simulink model "RotaryPendulum_SLdemo_SwingUp"  (R2015a)
settings: Solver=ode45  StartTime=0.0  StopTime=30  MaxStep=1e-3
InitFcn:
  | RotaryPendulum_PARAM;
values from neighbouring files (symbols this model uses):
  R = 0    [RotaryPendulum_MLdemo.m]
undefined symbols (not defined in the file or in its folder): g, I, l, m
libraries: vrlib x1, aerolibanimutils x1
settings Model: CovSFcnEnable=off  Creator=mischak  LastModifiedBy=mischak
settings DebuggingCC: SolverPrmCheckMsg=warning

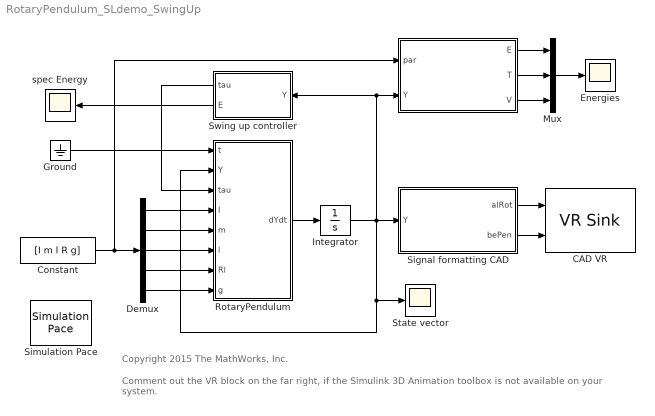
== system RotaryPendulum_SLdemo_SwingUp ==
  note: Comment out the VR block on the far right, if the Simulink 3D Animation toolbox is not available on your system.
  note: Copyright 2015 The MathWorks, Inc.
  " " : MATLAB Function  TreatAsAtomicUnit=on
  CAD VR : vrlib/VR Sink  InstantiateOnLoad=on  SampleTime=0.1  ViewEnable=on  RemoteChange=off  RemoteView=off  FieldsWritten=BFrame.rotation.4.1.1.double#EFrame.rotation.4.1.1.double  WorldFileName=SolidWorksS3D.wrl  AutoView=off  VideoDimensions=[]  AllowVariableSize=off  mask(Virtual Reality Sink){}
      mask Display: image(imread('SolidWorksS3D_icon.png'))
  Constant : Constant  Value=[I m l R g]
  Demux : Demux  Outputs=5
  Energies : Scope
      settings: YMin=-0.003  YMax=0.006
  Ground : Ground
  Integrator : Integrator  InitialCondition=[0 0 3.2 0.2]
  Mux : Mux  Inputs=3
  RotaryPendulum : MATLAB Function  TreatAsAtomicUnit=on
  Signal formatting CAD : MATLAB Function  TreatAsAtomicUnit=on
  Simulation Pace : aerolibanimutils/Simulation Pace  SimulationPace=0.75  SleepMode=MATLAB Thread  OutputPaceError=off  SampleTime=1/20
      settings: AttributesFormatString=%<SimulationPace> sec/sec
  State vector : Scope
      settings: YMin=-12.5  YMax=12.5
  Swing up controller : MATLAB Function  TreatAsAtomicUnit=on
  spec Energy : Scope
      settings: YMin=-2.1  YMax=-1.9  SaveName=ScopeData3
  wires:
  Integrator/1 -> Signal formatting CAD/1(Y), RotaryPendulum/2(Y), State vector/1, " "/2(Y), Swing up controller/1(Y)
  RotaryPendulum/1(dYdt) -> Integrator/1
  Demux/1 -> RotaryPendulum/4(I)
  Demux/3 -> RotaryPendulum/6(l)
  Demux/4 -> RotaryPendulum/7(Rl)
  Demux/5 -> RotaryPendulum/8(g)
  Constant/1 -> " "/1(par), Demux/1
  Ground/1 -> RotaryPendulum/1(t)
  " "/2(T) -> Mux/2
  " "/1(E) -> Mux/1
  " "/3(V) -> Mux/3
  Mux/1 -> Energies/1
  Demux/2 -> RotaryPendulum/5(m)
  Swing up controller/1(tau) -> RotaryPendulum/3(tau)
  Swing up controller/2(E) -> spec Energy/1
  Signal formatting CAD/1(alRot) -> CAD VR/1
  Signal formatting CAD/2(bePen) -> CAD VR/2

== matlab function RotaryPendulum_SLdemo_SwingUp/  ==
  data: par input; Y input; E output; T output; V output
function [E,T,V] = ComputeEnergies(par,Y)
%#codegen
al  = Y(1);
dal = Y(2);
be  = Y(3);
dbe = Y(4);

I   = par(1);
m   = par(2);
l   = par(3);
R   = par(4);
g   = par(5);

T   = I*dal.^2/2 + m/2*(R^2*dal.^2 + l^2*dal.^2.*sin(be).^2/3 + ...
        l^2*dbe.^2/4 - R*l*dal.*dbe.*cos(be)) + m*l^2*dbe.^2/24;
V   = m*g*l/2*cos(be);
E   = T + V;
end

== matlab function RotaryPendulum_SLdemo_SwingUp/RotaryPendulum ==
  data: t input; dYdt output; Y input; tau input; I input; m input; l input; Rl input; g input
function dYdt = RotaryPendulum_ODE(t,Y,tau,I,m,l,Rl,g)
%#codegen

%    This function was generated by the Symbolic Math Toolbox version 6.2.
%    10-Jun-2015 13:24:25

t4 = Y(3);
t2 = sin(t4);
t3 = Rl.^2;
t5 = cos(t4);
t6 = Y(4);
t7 = t5.^2;
t8 = Y(2);
t9 = l.^2;
t10 = I.*1.2e1;
t11 = m.*t3.*1.2e1;
t12 = t2.^2;
t13 = m.*t9.*t12.*4.0;
t14 = t10+t11+t13-m.*t3.*t7.*9.0;
t15 = 1.0./t14;
t16 = t8.^2;
t17 = t6.^2;
dYdt = [t8;...
        t15.*(tau.*1.2e1+Rl.*g.*m.*t2.*t5.*9.0-Rl.*l.*m.*t2.*t17.*6.0-m.*t2.*t5.*t6.*t8.*t9.*8.0+Rl.*l.*m.*t2.*t7.*t16.*6.0);...
        t6;...
       (t15.*(I.*g.*t2.*1.8e1+Rl.*t5.*tau.*1.8e1+g.*m.*t2.*t3.*1.8e1+I.*l.*t2.*t5.*t16.*1.2e1+g.*m.*t2.*t9.*t12.*6.0+l.*m.*t2.*t3.*t5.*t16.*1.2e1-l.*m.*t2.*t3.*t5.*t17.*9.0-Rl.*m.*t2.*t6.*t7.*t8.*t9.*1.2e1+l.*m.*t2.*t5.*t9.*t12.*t16.*4.0))./l];

== matlab function RotaryPendulum_SLdemo_SwingUp/Swing up controller ==
  data: Y input; tau output; E output
function [tau,E] = Controller(Y)

be  = Y(3);
dbe = Y(4);

m = 3.3e-3;
l = 183.2e-3;
M = 20.3e-3;
R = 109e-3;
g = 9.81;

me    = 0.012;
re    = 0.02;
ma    = M - me;
Ino_e = ma*R^2/3;        % corrected I without encoder
Itot  = Ino_e + me*re^2; % corrected I with encoder
I     = Itot;

T   = m*l^2*dbe.^2/6;
V   = m*g*l/2*(cos(be) - 1);
k   = 2e-4;
E   = -V/(m*g*l/2);
KM  = -[-0.6546041454298,-0.227420998980632,21.721030694302865,1.751613999320421];

if (cos(be) < cosd(25))
    taum = 0.016;
    tau = min(+taum, max(-taum,k*E*sign(dbe*cos(be))));
else
    tau = KM*Y;
end

== matlab function RotaryPendulum_SLdemo_SwingUp/Signal formatting CAD ==
  data: alRot output; bePen output; Y input
function [alRot, bePen] = FormatOUT(Y)
al    = Y(1);
dal   = Y(2);
be    = Y(3);
dbe   = Y(4);


alRot = [0; 0; 1; al];
bePen = [1; 0; 0; be];
end
